simulink model "inverter"  (R2021b)
settings: Solver=VariableStepAuto  StartTime=0.0  StopTime=1  RelTol=1e-3
libraries: spsMosfetLib x4, spsDCVoltageSourceLib x1, spsSeriesRLCBranchLib x1, spsVoltageMeasurementLib x1, spspowerguiLib x1
settings Model: Creator=eee  LastModifiedBy=eee

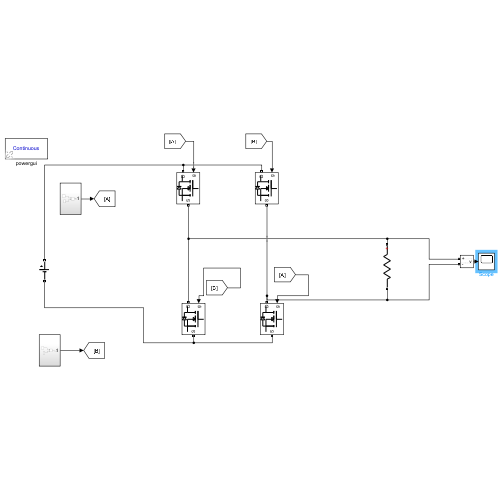
[thumbnail: Simulink's stored preview of the top-level diagram]
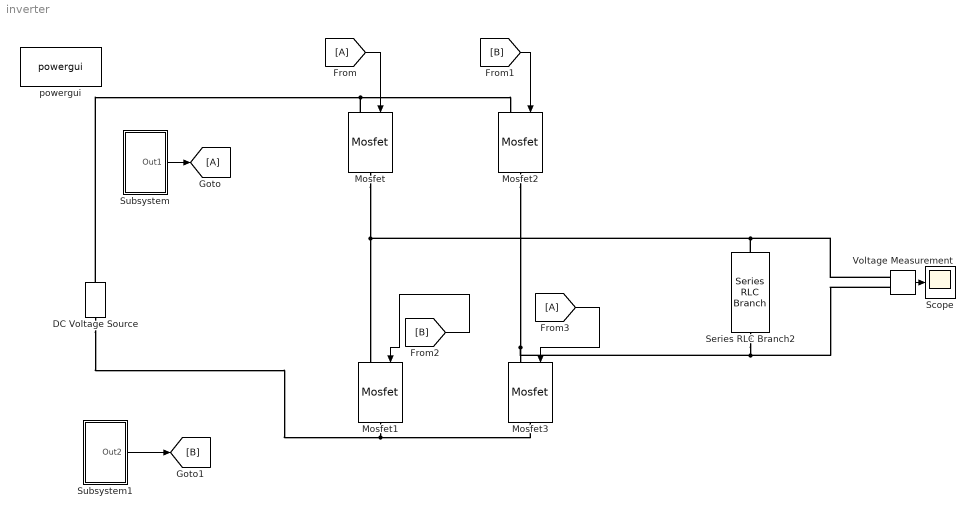
== system inverter ==
  DC Voltage Source : spsDCVoltageSourceLib/DC Voltage Source  Amplitude=100  Measurements=None
  Mosfet{,1..3} (4 alike) : spsMosfetLib/Mosfet  Ron=0.1  Lon=0  Rd=0.01  Vfd=0  IC=0  Rs=1e5  Cs=inf  Measurements=off
  Scope : Scope
  Series RLC Branch2 : spsSeriesRLCBranchLib/Series RLC Branch  LConnTagsString=__new0  RConnTagsString=__new0  BranchType=R  Resistance=100  Inductance=1e-3  SetiL0=off  InitialCurrent=0  Capacitance=1e-6  Setx0=off  InitialVoltage=0  Measurements=None
  Subsystem : Subsystem
  Subsystem1 : Subsystem
  Voltage Measurement : spsVoltageMeasurementLib/Voltage Measurement  PhasorSimulation=off  OutputType=Complex  PSBequivalent=0
  powergui : spspowerguiLib/powergui  Priority=1  SimulationMode=Continuous  SampleTime=50e-6  frequency=60  Iterations=50  frequencyindice=0  Pbase=100e6  ErrMax=1e-4  UnitsV=kV  UnitsW=MW  buscounter=0  FunctionMessages=off  echomessages=off  EnableUseOfTLC=off  CurrentSourceSwitches=off  DisableSnubberDevices=off  DisableRonSwitches=off  DisableVfSwitches=off  DisplayEquations=off  AutomaticDiscreteSolvers=off  SolverType=Tustin/Backward Euler (TBE)  Interpol=off  ExternalGateDelay=off  methode=off  Ts=100  x0status=blocks  SPID=on  SwTol=0  HookPort=off  NonlinearTolerance=1e-4  nMaxIteration=100  ContinueOnMaxIteration=off  RestoreLinks=warning  ResistiveCurrentMeasurement=off  Frange=[0:2:500]  Ylog=off  Xlog=on  ShowGrid=off  save=off  variable=ZData  structure=0  ZoomFFT=off  StartTime=0.0  cycles=1  DisplayStyle=1  fundamental=60  FreqAxis=off  MaxFrequency=1000  frequencyindicesteady=1  RmsSteady=1  display=off
  wires:
  Voltage Measurement/1 -> Scope/1
  [B] -> Mosfet1/1
  [B] -> Mosfet2/1
  [A] -> Mosfet3/1
  Subsystem/1(Out1) -> [A]
  Subsystem1/1(Out2) -> [B]
  [A] -> Mosfet/1
  connections:
  Mosfet2/RConn1 -- Voltage Measurement/LConn2 -- Series RLC Branch2/RConn1 -- Mosfet3/LConn1
  Mosfet/RConn1 -- Voltage Measurement/LConn1 -- Series RLC Branch2/LConn1 -- Mosfet1/LConn1
  Mosfet/LConn1 -- Mosfet2/LConn1 -- DC Voltage Source/RConn1
  Mosfet1/RConn1 -- Mosfet3/RConn1 -- DC Voltage Source/LConn1

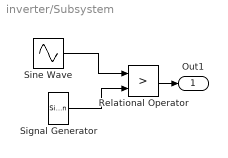
== system inverter/Subsystem ==
  Relational Operator : RelationalOperator  Operator=>  OutDataTypeStr=boolean  RndMeth=Simplest
  Signal Generator : SignalGenerator  WaveForm=sawtooth  Frequency=20000
  Sine Wave : Sin  Amplitude=.9  Frequency=2*pi*50  SampleTime=0
  Out1 : Outport
  wires:
  Signal Generator/1 -> Relational Operator/2
  Sine Wave/1 -> Relational Operator/1
  Relational Operator/1 -> Out1/1

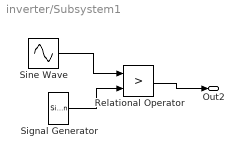
== system inverter/Subsystem1 ==
  Relational Operator : RelationalOperator  Operator=>  OutDataTypeStr=boolean  RndMeth=Simplest
  Signal Generator : SignalGenerator  WaveForm=sawtooth  Frequency=20000
  Sine Wave : Sin  Amplitude=0.9  Frequency=2*pi*50  Phase=pi  SampleTime=0
  Out2 : Outport
  wires:
  Sine Wave/1 -> Relational Operator/1
  Signal Generator/1 -> Relational Operator/2
  Relational Operator/1 -> Out2/1
